simulink model "PCS_pu_DCDC"  (R2024a)
settings: Solver=FixedStepAuto  StartTime=0.0  StopTime=3  RelTol=1e-3
undefined symbols (not defined in the file or in its folder): DiscIntNeverNeededParam, initial
libraries: spsCurrentMeasurementLib x18, spsVoltageMeasurementLib x13, spsControlledVoltageSourceLib x9, spsSeriesRLCBranchLib x7, spsThreePhaseSeriesRLCBranchLib x5, slpidlib x4, spsGroundLib x2, spsControlledCurrentSourceLib x2, SimplusGT x2, spspowerguiLib x2
(part 2 of 2)

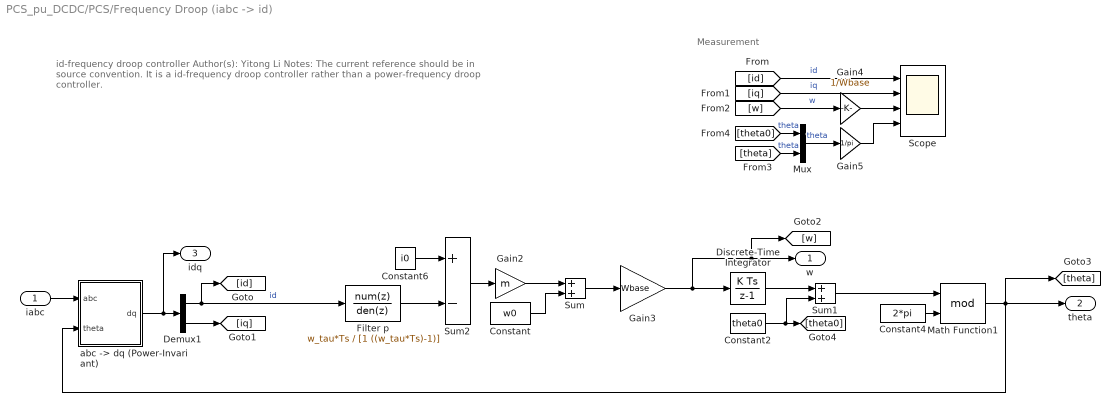
== system PCS_pu_DCDC/PCS/Frequency Droop (iabc -> id) ==
  note: Measurement
  note: id-frequency droop controller
      |
      | Author(s): Yitong Li
      |
      | Notes:
      |
      | The current reference should be in source convention.
      |
      | It is a id-frequency droop controller rather than a power-frequency droop controller.
  iabc : Inport
  Constant : Constant  Value=w0
  Constant2 : Constant  Value=theta0
  Constant4 : Constant  Value=2*pi
  Constant6 : Constant  Value=i0
  Demux1 : Demux  Outputs=2
  Discrete-Time Integrator : DiscreteIntegrator  SampleTime=Ts  ICPrevOutput=DiscIntNeverNeededParam  ICPrevScaledInput=DiscIntNeverNeededParam
  Filter p : DiscreteTransferFcn  Numerator=w_tau*Ts  Denominator=[1 ((w_tau*Ts)-1)]  SampleTime=Ts
  Gain2 : Gain  Gain=m
  Gain3 : Gain  Gain=Wbase
  Gain4 : Gain  Gain=1/Wbase
  Gain5 : Gain  Gain=1/pi
  Math Function1 : Math  Operator=mod  SignedPower=on
  Mux : Mux  Inputs=2
  Scope : Scope  NumInputPorts=4
  Sum : Sum
  Sum1 : Sum
  Sum2 : Sum  Inputs=+-
  "abc -> dq (Power-Invariant)" : Subsystem  AncestorBlock=|
      | SimplusGT/abc -> dq
      | (Power-Invariant)
  w : Outport
  theta : Outport  Port=2
  idq : Outport  Port=3
  wires:
  Sum1/1 -> Math Function1/1
  Constant2/1 -> Sum1/2, [theta0]
  Math Function1/1 -> "abc -> dq (Power-Invariant)"/2(theta), [theta], theta/1
  Gain2/1 -> Sum/1
  Discrete-Time Integrator/1 -> Sum1/1
  Filter p/1 -> Sum2/2
  Constant/1 -> Sum/2
  "abc -> dq (Power-Invariant)"/1(dq) -> idq/1, Demux1/1
  Constant4/1 -> Math Function1/2
  iabc/1 -> "abc -> dq (Power-Invariant)"/1(abc)
  Constant6/1 -> Sum2/1
  Sum2/1 -> Gain2/1
  Sum/1 -> Gain3/1
  Gain3/1 -> [w], w/1, Discrete-Time Integrator/1
  Demux1/1 -> [id], Filter p/1  "id"
  Gain5/1 -> Scope/4
  [iq] -> Scope/2  "iq"
  [theta0] -> Mux/1  "theta"
  [id] -> Scope/1  "id"
  Mux/1 -> Gain5/1  "theta"
  [theta] -> Mux/2  "theta"
  Demux1/2 -> [iq]
  [w] -> Gain4/1  "w"
  Gain4/1 -> Scope/3

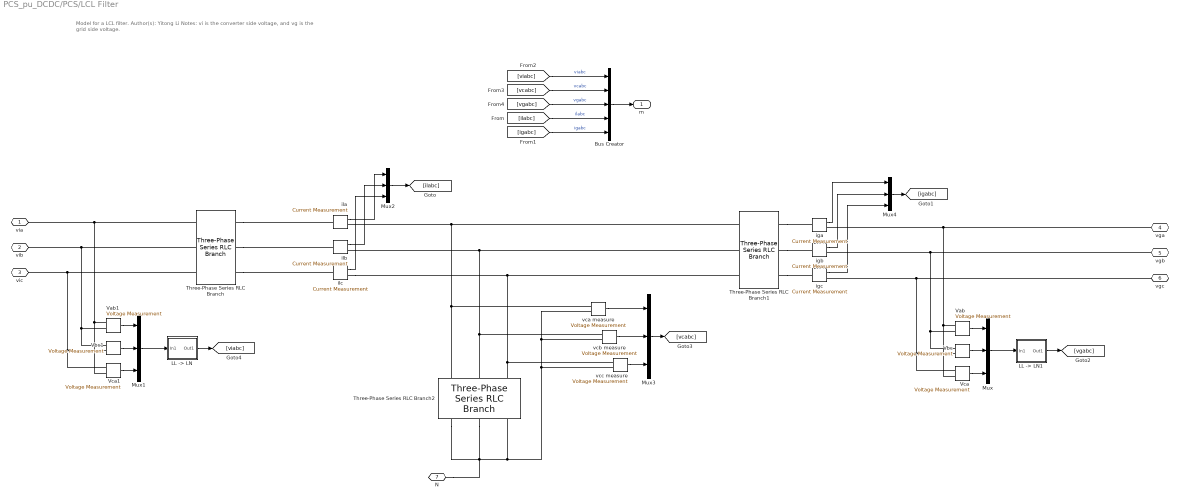
== system PCS_pu_DCDC/PCS/LCL Filter ==
  note: Model for a LCL filter.
      |
      | Author(s): Yitong Li
      |
      | Notes:
      |
      | vi is the converter side voltage, and vg is the grid side voltage.
  Bus Creator : BusCreator  Inputs=5
  "LL -> LN" : Subsystem  AncestorBlock=SimplusGT/LL -> LN
  "LL -> LN1" : Subsystem  AncestorBlock=|
      | SimplusGT/Grid-Forming Inverter
      | (Simulink Block)/LCL Filter/LL -> LN
  Mux{,1..4} (5 alike) : Mux  Inputs=3
  Three-Phase Series RLC Branch : spsThreePhaseSeriesRLCBranchLib/Three-Phase Series RLC Branch  LConnTagsString=A|B|C  RConnTagsString=A|B|C  BranchType=RL  Resistance=Rf  Inductance=Lf  Capacitance=1e-6  Measurements=None
  Three-Phase Series RLC Branch1 : spsThreePhaseSeriesRLCBranchLib/Three-Phase Series RLC Branch  LConnTagsString=A|B|C  RConnTagsString=A|B|C  BranchType=RL  Resistance=Rc  Inductance=Lc  Capacitance=1e-6  Measurements=None
  Three-Phase Series RLC Branch2 : spsThreePhaseSeriesRLCBranchLib/Three-Phase Series RLC Branch  LConnTagsString=A|B|C  RConnTagsString=A|B|C  BranchType=RC  Resistance=Rd  Inductance=Lc  Capacitance=Cf  Measurements=None
  Vab : spsVoltageMeasurementLib/Voltage Measurement  PhasorSimulation=off  OutputType=Complex  PSBequivalent=0
  Vab1 : spsVoltageMeasurementLib/Voltage Measurement  PhasorSimulation=off  OutputType=Complex  PSBequivalent=0
  Vbc : spsVoltageMeasurementLib/Voltage Measurement  PhasorSimulation=off  OutputType=Complex  PSBequivalent=0
  Vbc1 : spsVoltageMeasurementLib/Voltage Measurement  PhasorSimulation=off  OutputType=Complex  PSBequivalent=0
  Vca : spsVoltageMeasurementLib/Voltage Measurement  PhasorSimulation=off  OutputType=Complex  PSBequivalent=0
  Vca1 : spsVoltageMeasurementLib/Voltage Measurement  PhasorSimulation=off  OutputType=Complex  PSBequivalent=0
  iga : spsCurrentMeasurementLib/Current Measurement  PhasorSimulation=off  OutputType=Complex  PSBequivalent=0
  igb : spsCurrentMeasurementLib/Current Measurement  PhasorSimulation=off  OutputType=Complex  PSBequivalent=0
  igc : spsCurrentMeasurementLib/Current Measurement  PhasorSimulation=off  OutputType=Complex  PSBequivalent=0
  ila : spsCurrentMeasurementLib/Current Measurement  PhasorSimulation=off  OutputType=Complex  PSBequivalent=0
  ilb : spsCurrentMeasurementLib/Current Measurement  PhasorSimulation=off  OutputType=Complex  PSBequivalent=0
  ilc : spsCurrentMeasurementLib/Current Measurement  PhasorSimulation=off  OutputType=Complex  PSBequivalent=0
  vca measure : spsVoltageMeasurementLib/Voltage Measurement  PhasorSimulation=off  OutputType=Complex  PSBequivalent=0
  vcb measure : spsVoltageMeasurementLib/Voltage Measurement  PhasorSimulation=off  OutputType=Complex  PSBequivalent=0
  vcc measure : spsVoltageMeasurementLib/Voltage Measurement  PhasorSimulation=off  OutputType=Complex  PSBequivalent=0
  via : PMIOPort  Side=Left
  vib : PMIOPort  Port=2  Side=Left
  vic : PMIOPort  Port=3  Side=Left
  vga : PMIOPort  Port=4  Side=Right
  vgb : PMIOPort  Port=5  Side=Right
  vgc : PMIOPort  Port=6  Side=Right
  N : PMIOPort  Port=7  Side=Left
  m : Outport
  wires:
  Mux4/1 -> [igabc]
  ilb/1 -> Mux2/2
  ila/1 -> Mux2/1
  igc/1 -> Mux4/3
  vcc measure/1 -> Mux3/3
  Vab/1 -> Mux/1
  Mux/1 -> "LL -> LN1"/1(In1)
  vca measure/1 -> Mux3/1
  vcb measure/1 -> Mux3/2
  igb/1 -> Mux4/2
  iga/1 -> Mux4/1
  Vca/1 -> Mux/3
  ilc/1 -> Mux2/3
  Vbc/1 -> Mux/2
  Mux2/1 -> [ilabc]
  Bus Creator/1 -> m/1
  "LL -> LN1"/1(Out1) -> [vgabc]
  Mux3/1 -> [vcabc]
  Vbc1/1 -> Mux1/2
  Vca1/1 -> Mux1/3
  Mux1/1 -> "LL -> LN"/1(In1)
  Vab1/1 -> Mux1/1
  "LL -> LN"/1(Out1) -> [viabc]
  [viabc] -> Bus Creator/1  "viabc"
  [vcabc] -> Bus Creator/2  "vcabc"
  [vgabc] -> Bus Creator/3  "vgabc"
  [ilabc] -> Bus Creator/4  "ilabc"
  [igabc] -> Bus Creator/5  "igabc"
  connections:
  Three-Phase Series RLC Branch2/RConn1 -- Three-Phase Series RLC Branch2/RConn2 -- N/RConn1 -- Three-Phase Series RLC Branch2/RConn3 -- vcc measure/LConn2 -- vca measure/LConn2 -- vcb measure/LConn2
  Vca/LConn1 -- Vbc/LConn2 -- igc/RConn1 -- vgc/RConn1
  Vca1/LConn1 -- Vbc1/LConn2 -- vic/RConn1 -- Three-Phase Series RLC Branch/LConn3
  Three-Phase Series RLC Branch/LConn2 -- Vbc1/LConn1 -- Vab1/LConn2 -- vib/RConn1
  Vab1/LConn1 -- Vca1/LConn2 -- via/RConn1 -- Three-Phase Series RLC Branch/LConn1
  Three-Phase Series RLC Branch1/LConn3 -- ilc/RConn1 -- Three-Phase Series RLC Branch2/LConn3 -- vcc measure/LConn1
  Three-Phase Series RLC Branch1/RConn2 -- igb/LConn1
  Vbc/LConn1 -- Vab/LConn2 -- igb/RConn1 -- vgb/RConn1
  ilb/RConn1 -- Three-Phase Series RLC Branch1/LConn2 -- vcb measure/LConn1 -- Three-Phase Series RLC Branch2/LConn2
  ila/RConn1 -- Three-Phase Series RLC Branch1/LConn1 -- vca measure/LConn1 -- Three-Phase Series RLC Branch2/LConn1
  Vab/LConn1 -- Vca/LConn2 -- iga/RConn1 -- vga/RConn1
  Three-Phase Series RLC Branch1/RConn1 -- iga/LConn1
  Three-Phase Series RLC Branch1/RConn3 -- igc/LConn1
  Three-Phase Series RLC Branch/RConn1 -- ila/LConn1
  Three-Phase Series RLC Branch/RConn2 -- ilb/LConn1
  Three-Phase Series RLC Branch/RConn3 -- ilc/LConn1

== system PCS_pu_DCDC/PCS/PQ Calculation (dq-Frame) ==
  note: Power calculation.
      |
      | Author(s): Yitong Li
      |
      | Notes:
      |
      | The calculation is done in dq frame.
  vdq : Inport
  idq : Inport  Port=2
  Mux : Mux  Inputs=2
  Mux1 : Mux  Inputs=2
  P = vd*id+vq*iq : Fcn  Expr=u[1]*u[3]+u[2]*u[4]
  Q = -vd*iq+vq*id : Fcn  Expr=-u[1]*u[4]+u[2]*u[3]
  pq : Outport
  wires:
  Q = -vd*iq+vq*id/1 -> Mux/2
  Mux1/1 -> Q = -vd*iq+vq*id/1, P = vd*id+vq*iq/1
  idq/1 -> Mux1/2
  vdq/1 -> Mux1/1
  P = vd*id+vq*iq/1 -> Mux/1
  Mux/1 -> pq/1

== system PCS_pu_DCDC/PCS/SC_Voltage_controller ==
  vdc : Inport
  vdc_ref : Inport  Port=2
  Add : Sum  Inputs=+-
  Discrete PID Controller : slpidlib/PID Controller  Controller=PID  Form=Parallel  TimeDomain=Discrete-time  UseExternalTs=off  SampleTime=-1  IntegratorMethod=Forward Euler  FilterMethod=Forward Euler  ControllerParametersSource=internal  P=w_v*C  I=w_v*w_v*C/4  UseKiTs=off  D=0  UseExternalDerivativeSource=off  N=100  UseFilter=off  TunerSelectOption=Transfer Function Based (PID Tuner App)  InitialConditionSource=internal  InitialConditionForIntegrator=0  InitialConditionForFilter=0  DifferentiatorICPrevScaledInput=0  ExternalReset=none  TrackingMode=off  Kt=1  LimitOutput=off  SatLimitsSource=internal  UpperSaturationLimit=inf  LowerSaturationLimit=-inf  LinearizeAsGain=off  AntiWindupMode=none  Kb=1  LimitIntegrator=off  UpperIntegratorSaturationLimit=inf  LowerIntegratorSaturationLimit=-inf  POutMin=[]  POutMax=[]  IOutMin=[]  IOutMax=[]  DOutMin=[]  DOutMax=[]  NOutMin=[]  NOutMax=[]  SumOutMin=[]  SumOutMax=[]  SaturationOutMin=[]  SaturationOutMax=[]  PParamMin=[]  PParamMax=[]  IParamMin=[]  IParamMax=[]  DParamMin=[]  DParamMax=[]  NParamMin=[]  NParamMax=[]  KbParamMin=[]  KbParamMax=[]  KtParamMin=[]  KtParamMax=[]  KbOutMin=[]  KbOutMax=[]  KtOutMin=[]  KtOutMax=[]  IntegratorOutMin=[]  IntegratorOutMax=[]  FilterOutMin=[]  FilterOutMax=[]  SumI1OutMin=[]  SumI1OutMax=[]  SumI2OutMin=[]  SumI2OutMax=[]  SumI3OutMin=[]  SumI3OutMax=[]  SumI4OutMin=[]  SumI4OutMax=[]  SumDOutMin=[]  SumDOutMax=[]  DifferentiatorOutMin=[]  DifferentiatorOutMax=[]  FilterDiffOutCoefMin=[]  FilterDiffOutCoefMax=[]  ReciprocalOutMin=[]  ReciprocalOutMax=[]  SumDenOutMin=[]  SumDenOutMax=[]  SumNumOutMin=[]  SumNumOutMax=[]  DivideOutMin=[]  DivideOutMax=[]  UdiffTsProdOutMin=[]  UdiffTsProdOutMax=[]  NTsProdOutMin=[]  NTsProdOutMax=[]  UintegralTsProdOutMin=[]  UintegralTsProdOutMax=[]  UngainTsProdOutMin=[]  UngainTsProdOutMax=[]  ClampingZeroOutDataTypeStr=Inherit: Inherit via back propagation  ClampingZeroOutMin=[]  ClampingZeroOutMax=[]  FilterDenConstantOutDataTypeStr=Inherit: Inherit via back propagation  FilterDenConstantOutMin=[]  FilterDenConstantOutMax=[]  PCopyOutDataTypeStr=Inherit: Inherit via back propagation  PCopyOutMin=[]  PCopyOutMax=[]  NCopyOutDataTypeStr=Inherit: Inherit via back propagation  NCopyOutMin=[]  NCopyOutMax=[]  IntegratorContinuousStateAttributes=''  IntegratorStateMustResolveToSignalObject=off  IntegratorRTWStateStorageClass=Auto  FilterContinuousStateAttributes=''  FilterStateMustResolveToSignalObject=off  FilterRTWStateStorageClass=Auto  ParallelPVariant=InternalParameters  IdealPVariant=Disabled  IVariant=InternalParameters  DVariant=InternalParameters  IntegratorVariant=Discrete  SatVariant=Disabled  AWVariant=Passthrough  PCopyVariant=Disabled  TRVariant=Disabled  FdbkBlocksVariant=Forward  IdealPFdbkVariant=Disabled  SatFdbkVariant=Disabled  DerivativeFilterVariant=Differentiator  NVariant=Passthrough  NCopyVariant=Disabled_SignalSpec  FilterICVariant=InternalICsDifferentiator  IntegratorICVariant=InternalICs  ExternalResetVariant=Disabled  TRSumVariant=Passthrough  SumFdbkVariant=Disabled  SumVariant=Sum_PID  TsampFilterVariant=InternalTs  TsampNgainVariant=Passthrough  TsampIntegralVariant=Disabled_SignalSpec  ExternalSaturationOutDataTypeStr=Inherit: Same as second input  DerivativeSourceVariant=ErrorSignal
      settings: LibrarySourceBlock=simulink/Discrete/Discrete PID Controller
  Display : Display
  Display1 : Display
  i_ref : Outport
  wires:
  vdc_ref/1 -> Add/1
  vdc/1 -> Add/2
  Add/1 -> Display/1, Discrete PID Controller/1
  Discrete PID Controller/1 -> Display1/1, i_ref/1

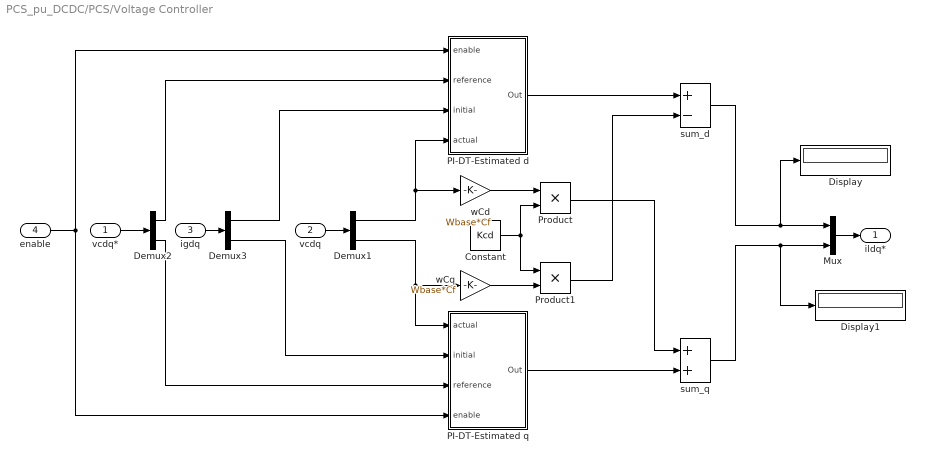
== system PCS_pu_DCDC/PCS/Voltage Controller ==
  vcdq* : Inport
  vcdq : Inport  Port=2
  igdq : Inport  Port=3
  enable : Inport  Port=4
  Constant : Constant  Value=Kcd
  Demux1 : Demux  Outputs=2
  Demux2 : Demux  Outputs=2
  Demux3 : Demux  Outputs=2
  Display : Display
  Display1 : Display
  Mux : Mux  Inputs=2
  PI-DT-Estimated d : Subsystem  mask{Kg=Kg, Kp=Kp, Ki=Ki, xmax=xdmax, xmin=-xdmax, Ts=Ts}
      mask prompts: Kg "Estimator Gain"; Kp "Proportional Gain"; Ki "Integral Gain"; xmax "Upper Limit"; xmin "Lower Limit"; Ts "Sampling Time"
  PI-DT-Estimated q : Subsystem  mask{Kg=Kg, Kp=Kp, Ki=Ki, xmax=xqmax, xmin=-xqmax, Ts=Ts}
      mask prompts: Kg "Estimator Gain"; Kp "Proportional Gain"; Ki "Integral Gain"; xmax "Upper Limit"; xmin "Lower Limit"; Ts "Sampling Time"
  Product : Product
  Product1 : Product
  sum_d : Sum  Inputs=+-
  sum_q : Sum
  wCd : Gain  Gain=Wbase*Cf
  wCq : Gain  Gain=Wbase*Cf
  ildq* : Outport
  wires:
  Constant/1 -> Product1/1, Product/2
  Product1/1 -> sum_d/2
  wCq/1 -> Product1/2
  Product/1 -> sum_q/1
  wCd/1 -> Product/1
  enable/1 -> PI-DT-Estimated d/1(enable), PI-DT-Estimated q/4(enable)
  Demux2/2 -> PI-DT-Estimated q/3(reference)
  Demux2/1 -> PI-DT-Estimated d/2(reference)
  vcdq*/1 -> Demux2/1
  Demux3/1 -> PI-DT-Estimated d/3(initial)
  Demux3/2 -> PI-DT-Estimated q/2(initial)
  PI-DT-Estimated q/1(Out) -> sum_q/2
  igdq/1 -> Demux3/1
  PI-DT-Estimated d/1(Out) -> sum_d/1
  Mux/1 -> ildq*/1
  Demux1/2 -> wCq/1, PI-DT-Estimated q/1(actual)
  Demux1/1 -> PI-DT-Estimated d/4(actual), wCd/1
  vcdq/1 -> Demux1/1
  sum_q/1 -> Display1/1, Mux/2
  sum_d/1 -> Display/1, Mux/1

== system PCS_pu_DCDC/PCS/abc -> dq (Power-Invariant) ==
  note: Frame transformation from abc to dq.
      |
      | Author(s): Yitong Li
      |
      | Notes:
      |
      | The transformation is power-invariant.
      |
      | theta is the angle that d axis leads a axis.
      |
      | q axis leads d axis by 90 degrees.
  abc : Inport
  theta : Inport  Port=2
  ->d : Fcn  Expr=cos(u(4))*u(1) + cos(u(4)-2/3*pi)*u(2) + cos(u(4)-4/3*pi)*u(3)
  ->q : Fcn  Expr=-sin(u(4))*u(1) - sin(u(4)-2/3*pi)*u(2) - sin(u(4)-4/3*pi)*u(3)
  Gain : Gain  Gain=sqrt(2/3)
  Mux5 : Mux  Inputs=2
  Mux6 : Mux  Inputs=2
  dq : Outport
  wires:
  Mux5/1 -> ->q/1, ->d/1
  Mux6/1 -> dq/1
  ->q/1 -> Mux6/2
  theta/1 -> Mux5/2
  Gain/1 -> Mux5/1
  ->d/1 -> Mux6/1
  abc/1 -> Gain/1

== system PCS_pu_DCDC/PCS/abc -> dq (Power-Invariant)1 ==
  note: Frame transformation from abc to dq.
      |
      | Author(s): Yitong Li
      |
      | Notes:
      |
      | The transformation is power-invariant.
      |
      | theta is the angle that d axis leads a axis.
      |
      | q axis leads d axis by 90 degrees.
  abc : Inport
  theta : Inport  Port=2
  ->d : Fcn  Expr=cos(u(4))*u(1) + cos(u(4)-2/3*pi)*u(2) + cos(u(4)-4/3*pi)*u(3)
  ->q : Fcn  Expr=-sin(u(4))*u(1) - sin(u(4)-2/3*pi)*u(2) - sin(u(4)-4/3*pi)*u(3)
  Gain : Gain  Gain=sqrt(2/3)
  Mux5 : Mux  Inputs=2
  Mux6 : Mux  Inputs=2
  dq : Outport
  wires:
  Mux5/1 -> ->q/1, ->d/1
  Mux6/1 -> dq/1
  ->q/1 -> Mux6/2
  theta/1 -> Mux5/2
  Gain/1 -> Mux5/1
  ->d/1 -> Mux6/1
  abc/1 -> Gain/1

== system PCS_pu_DCDC/PCS/abc -> dq (Power-Invariant)2 ==
  note: Frame transformation from abc to dq.
      |
      | Author(s): Yitong Li
      |
      | Notes:
      |
      | The transformation is power-invariant.
      |
      | theta is the angle that d axis leads a axis.
      |
      | q axis leads d axis by 90 degrees.
  abc : Inport
  theta : Inport  Port=2
  ->d : Fcn  Expr=cos(u(4))*u(1) + cos(u(4)-2/3*pi)*u(2) + cos(u(4)-4/3*pi)*u(3)
  ->q : Fcn  Expr=-sin(u(4))*u(1) - sin(u(4)-2/3*pi)*u(2) - sin(u(4)-4/3*pi)*u(3)
  Gain : Gain  Gain=sqrt(2/3)
  Mux5 : Mux  Inputs=2
  Mux6 : Mux  Inputs=2
  dq : Outport
  wires:
  Mux5/1 -> ->q/1, ->d/1
  Mux6/1 -> dq/1
  ->q/1 -> Mux6/2
  theta/1 -> Mux5/2
  Gain/1 -> Mux5/1
  ->d/1 -> Mux6/1
  abc/1 -> Gain/1

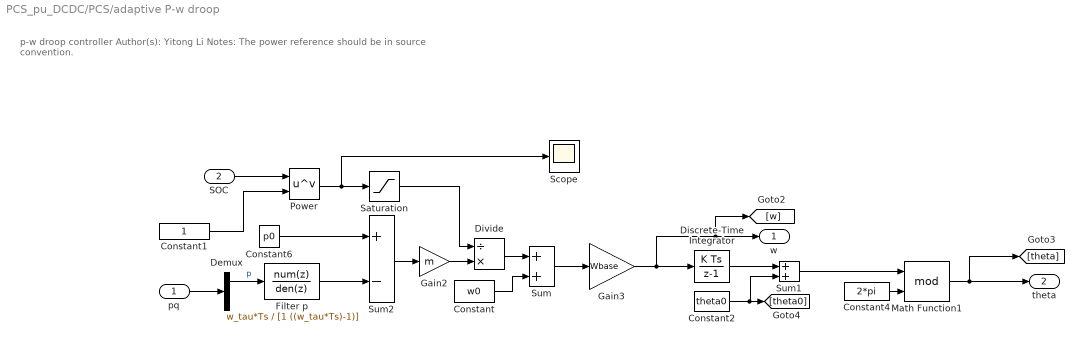
== system PCS_pu_DCDC/PCS/adaptive P-w droop ==
  note: p-w droop controller
      |
      | Author(s): Yitong Li
      |
      | Notes:
      |
      | The power reference should be in source convention.
  pq : Inport
  SOC : Inport  Port=2
  Constant : Constant  Value=w0
  Constant1 : Constant
  Constant2 : Constant  Value=theta0
  Constant4 : Constant  Value=2*pi
  Constant6 : Constant  Value=p0
  Demux : Demux  Outputs=2
  Discrete-Time Integrator : DiscreteIntegrator  SampleTime=Ts  ICPrevOutput=DiscIntNeverNeededParam  ICPrevScaledInput=DiscIntNeverNeededParam
  Divide : Product  Inputs=/*
  Filter p : DiscreteTransferFcn  Numerator=w_tau*Ts  Denominator=[1 ((w_tau*Ts)-1)]  SampleTime=Ts
  Gain2 : Gain  Gain=m
  Gain3 : Gain  Gain=Wbase
  Math Function1 : Math  Operator=mod  SignedPower=on
  Power : Math  Operator=pow
  Saturation : Saturate  UpperLimit=1  LowerLimit=0.1
  Scope : Scope
  Sum : Sum
  Sum1 : Sum
  Sum2 : Sum  Inputs=+-
  w : Outport
  theta : Outport  Port=2
  wires:
  Demux/1 -> Filter p/1  "p"
  Sum1/1 -> Math Function1/1
  Constant2/1 -> Sum1/2, [theta0]
  Math Function1/1 -> [theta], theta/1
  Discrete-Time Integrator/1 -> Sum1/1
  Filter p/1 -> Sum2/2
  Constant/1 -> Sum/2
  Constant4/1 -> Math Function1/2
  pq/1 -> Demux/1
  Constant6/1 -> Sum2/1
  Sum2/1 -> Gain2/1
  Sum/1 -> Gain3/1
  Gain3/1 -> [w], w/1, Discrete-Time Integrator/1
  Gain2/1 -> Divide/2
  Divide/1 -> Sum/1
  Saturation/1 -> Divide/1
  SOC/1 -> Power/1
  Power/1 -> Scope/1, Saturation/1
  Constant1/1 -> Power/2

== system PCS_pu_DCDC/PCS/dq -> abc (Power-Invariant) ==
  note: Frame transformation from dq to abc.
      |
      | Author(s): Yitong Li
      |
      | Notes:
      |
      | The transformation is power-invariant.
      |
      | theta is the angle that dq axis leads alpha/beta axis, specifically, d axis leads alpha axis.
  dq : Inport
  theta : Inport  Port=2
  ->a : Fcn  Expr=cos(u(3))*u(1) - sin(u(3))*u(2)
  ->b : Fcn  Expr=cos(u(3)-2/3*pi)*u(1) - sin(u(3)-2/3*pi)*u(2)
  ->c : Fcn  Expr=cos(u(3)-4/3*pi)*u(1) - sin(u(3)-4/3*pi)*u(2)
  Gain : Gain  Gain=sqrt(2/3)
  Mux5 : Mux  Inputs=2
  Mux6 : Mux  Inputs=3
  abc : Outport
  wires:
  theta/1 -> Mux5/2
  Mux5/1 -> ->c/1, ->a/1, ->b/1
  Mux6/1 -> abc/1
  ->c/1 -> Mux6/3
  dq/1 -> Gain/1
  Gain/1 -> Mux5/1
  ->a/1 -> Mux6/1
  ->b/1 -> Mux6/2

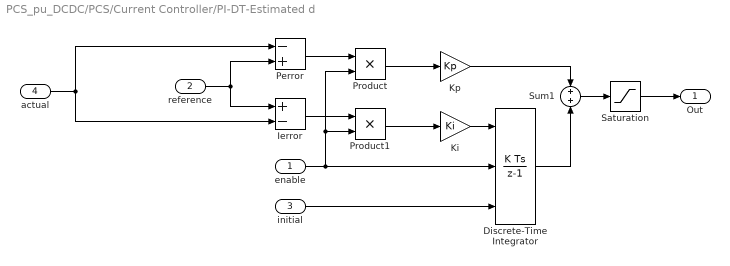
== system PCS_pu_DCDC/PCS/Current Controller/PI-DT-Estimated d ==
  enable : Inport
  reference : Inport  Port=2
  initial : Inport  Port=3
  actual : Inport  Port=4
  Discrete-Time Integrator : DiscreteIntegrator  gainval=1  ExternalReset=rising  InitialConditionSource=external  InitialCondition=initial  SampleTime=Ts  LimitOutput=on  UpperSaturationLimit=xmax  LowerSaturationLimit=xmin  ICPrevOutput=DiscIntNeverNeededParam  ICPrevScaledInput=DiscIntNeverNeededParam
  Ierror : Sum  Inputs=+-
  Ki : Gain  Gain=Ki  SaturateOnIntegerOverflow=on  OutDataTypeStr=Inherit: Same as input  ParamDataTypeStr=Inherit: Same as input
  Kp : Gain  Gain=Kp  SaturateOnIntegerOverflow=on  OutDataTypeStr=Inherit: Same as input  ParamDataTypeStr=Inherit: Same as input
  Perror : Sum  Inputs=-+
  Product : Product  RndMeth=Zero
  Product1 : Product  RndMeth=Zero
  Saturation : Saturate  UpperLimit=xmax  LowerLimit=xmin
  Sum1 : Sum  SaturateOnIntegerOverflow=on
  Out : Outport
  wires:
  Product1/1 -> Ki/1
  Ierror/1 -> Product1/1
  Product/1 -> Kp/1
  Perror/1 -> Product/1
  reference/1 -> Ierror/1, Perror/2
  actual/1 -> Ierror/2, Perror/1
  initial/1 -> Discrete-Time Integrator/3
  enable/1 -> Product1/2, Product/2, Discrete-Time Integrator/2
  Discrete-Time Integrator/1 -> Sum1/2
  Kp/1 -> Sum1/1
  Ki/1 -> Discrete-Time Integrator/1
  Sum1/1 -> Saturation/1
  Saturation/1 -> Out/1

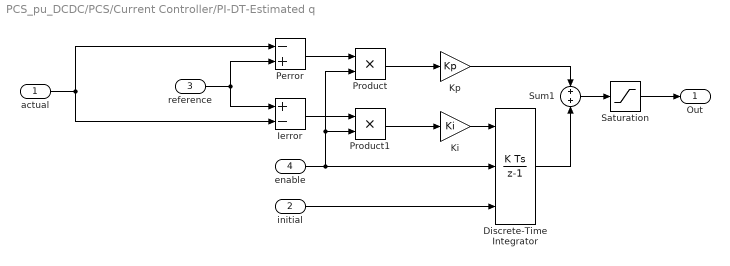
== system PCS_pu_DCDC/PCS/Current Controller/PI-DT-Estimated q ==
  actual : Inport
  initial : Inport  Port=2
  reference : Inport  Port=3
  enable : Inport  Port=4
  Discrete-Time Integrator : DiscreteIntegrator  gainval=1  ExternalReset=rising  InitialConditionSource=external  InitialCondition=initial  SampleTime=Ts  LimitOutput=on  UpperSaturationLimit=xmax  LowerSaturationLimit=xmin  ICPrevOutput=DiscIntNeverNeededParam  ICPrevScaledInput=DiscIntNeverNeededParam
  Ierror : Sum  Inputs=+-
  Ki : Gain  Gain=Ki  SaturateOnIntegerOverflow=on  OutDataTypeStr=Inherit: Same as input  ParamDataTypeStr=Inherit: Same as input
  Kp : Gain  Gain=Kp  SaturateOnIntegerOverflow=on  OutDataTypeStr=Inherit: Same as input  ParamDataTypeStr=Inherit: Same as input
  Perror : Sum  Inputs=-+
  Product : Product  RndMeth=Zero
  Product1 : Product  RndMeth=Zero
  Saturation : Saturate  UpperLimit=xmax  LowerLimit=xmin
  Sum1 : Sum  SaturateOnIntegerOverflow=on
  Out : Outport
  wires:
  Product1/1 -> Ki/1
  Ierror/1 -> Product1/1
  Product/1 -> Kp/1
  Perror/1 -> Product/1
  reference/1 -> Ierror/1, Perror/2
  actual/1 -> Perror/1, Ierror/2
  initial/1 -> Discrete-Time Integrator/3
  enable/1 -> Product1/2, Product/2, Discrete-Time Integrator/2
  Discrete-Time Integrator/1 -> Sum1/2
  Kp/1 -> Sum1/1
  Ki/1 -> Discrete-Time Integrator/1
  Sum1/1 -> Saturation/1
  Saturation/1 -> Out/1

== system PCS_pu_DCDC/PCS/Frequency Droop (iabc -> id)/abc -> dq (Power-Invariant) ==
  note: Frame transformation from abc to dq.
      |
      | Author(s): Yitong Li
      |
      | Notes:
      |
      | The transformation is power-invariant.
      |
      | theta is the angle that d axis leads a axis.
      |
      | q axis leads d axis by 90 degrees.
  abc : Inport
  theta : Inport  Port=2
  ->d : Fcn  Expr=cos(u(4))*u(1) + cos(u(4)-2/3*pi)*u(2) + cos(u(4)-4/3*pi)*u(3)
  ->q : Fcn  Expr=-sin(u(4))*u(1) - sin(u(4)-2/3*pi)*u(2) - sin(u(4)-4/3*pi)*u(3)
  Gain : Gain  Gain=sqrt(2/3)
  Mux5 : Mux  Inputs=2
  Mux6 : Mux  Inputs=2
  dq : Outport
  wires:
  abc/1 -> Gain/1
  ->d/1 -> Mux6/1
  Gain/1 -> Mux5/1
  theta/1 -> Mux5/2
  ->q/1 -> Mux6/2
  Mux6/1 -> dq/1
  Mux5/1 -> ->d/1, ->q/1

== system PCS_pu_DCDC/PCS/LCL Filter/LL -> LN ==
  note: Transformation from line-to-line voltage to line-to-neutral voltage.
      |
      | Author(s): Yitong Li
  In1 : Inport
  Fcn : Fcn  Expr=u[1]-u[3]
  Fcn1 : Fcn  Expr=u[2]-u[1]
  Fcn2 : Fcn  Expr=u[3]-u[2]
  Gain : Gain  Gain=1/3
  Mux9 : Mux  Inputs=3
  Out1 : Outport
  wires:
  In1/1 -> Gain/1
  Gain/1 -> Fcn/1, Fcn1/1, Fcn2/1
  Mux9/1 -> Out1/1
  Fcn2/1 -> Mux9/3
  Fcn1/1 -> Mux9/2
  Fcn/1 -> Mux9/1

== system PCS_pu_DCDC/PCS/LCL Filter/LL -> LN1 ==
  note: Transformation from line-to-line voltage to line-to-neutral voltage.
      |
      | Author(s): Yitong Li
  In1 : Inport
  Fcn : Fcn  Expr=u[1]-u[3]
  Fcn1 : Fcn  Expr=u[2]-u[1]
  Fcn2 : Fcn  Expr=u[3]-u[2]
  Gain : Gain  Gain=1/3
  Mux9 : Mux  Inputs=3
  Out1 : Outport
  wires:
  In1/1 -> Gain/1
  Gain/1 -> Fcn/1, Fcn1/1, Fcn2/1
  Mux9/1 -> Out1/1
  Fcn2/1 -> Mux9/3
  Fcn1/1 -> Mux9/2
  Fcn/1 -> Mux9/1

== system PCS_pu_DCDC/PCS/Voltage Controller/PI-DT-Estimated d ==
  enable : Inport
  reference : Inport  Port=2
  initial : Inport  Port=3
  actual : Inport  Port=4
  Discrete-Time Integrator : DiscreteIntegrator  gainval=1  ExternalReset=rising  InitialConditionSource=external  InitialCondition=initial  SampleTime=Ts  LimitOutput=on  UpperSaturationLimit=xmax  LowerSaturationLimit=xmin  ICPrevOutput=DiscIntNeverNeededParam  ICPrevScaledInput=DiscIntNeverNeededParam
  Ierror : Sum  Inputs=+-
  Ki : Gain  Gain=Ki  SaturateOnIntegerOverflow=on  OutDataTypeStr=Inherit: Same as input  ParamDataTypeStr=Inherit: Same as input
  Kp : Gain  Gain=Kp  SaturateOnIntegerOverflow=on  OutDataTypeStr=Inherit: Same as input  ParamDataTypeStr=Inherit: Same as input
  Perror : Sum  Inputs=-+
  Product : Product  RndMeth=Zero
  Product1 : Product  RndMeth=Zero
  Saturation : Saturate  UpperLimit=xmax  LowerLimit=xmin
  Sum1 : Sum  SaturateOnIntegerOverflow=on
  Out : Outport
  wires:
  Product1/1 -> Ki/1
  Ierror/1 -> Product1/1
  Product/1 -> Kp/1
  Perror/1 -> Product/1
  reference/1 -> Ierror/1, Perror/2
  actual/1 -> Ierror/2, Perror/1
  initial/1 -> Discrete-Time Integrator/3
  enable/1 -> Product1/2, Product/2, Discrete-Time Integrator/2
  Discrete-Time Integrator/1 -> Sum1/2
  Kp/1 -> Sum1/1
  Ki/1 -> Discrete-Time Integrator/1
  Sum1/1 -> Saturation/1
  Saturation/1 -> Out/1

== system PCS_pu_DCDC/PCS/Voltage Controller/PI-DT-Estimated q ==
  actual : Inport
  initial : Inport  Port=2
  reference : Inport  Port=3
  enable : Inport  Port=4
  Discrete-Time Integrator : DiscreteIntegrator  gainval=1  ExternalReset=rising  InitialConditionSource=external  InitialCondition=initial  SampleTime=Ts  LimitOutput=on  UpperSaturationLimit=xmax  LowerSaturationLimit=xmin  ICPrevOutput=DiscIntNeverNeededParam  ICPrevScaledInput=DiscIntNeverNeededParam
  Ierror : Sum  Inputs=+-
  Ki : Gain  Gain=Ki  SaturateOnIntegerOverflow=on  OutDataTypeStr=Inherit: Same as input  ParamDataTypeStr=Inherit: Same as input
  Kp : Gain  Gain=Kp  SaturateOnIntegerOverflow=on  OutDataTypeStr=Inherit: Same as input  ParamDataTypeStr=Inherit: Same as input
  Perror : Sum  Inputs=-+
  Product : Product  RndMeth=Zero
  Product1 : Product  RndMeth=Zero
  Saturation : Saturate  UpperLimit=xmax  LowerLimit=xmin
  Sum1 : Sum  SaturateOnIntegerOverflow=on
  Out : Outport
  wires:
  Product1/1 -> Ki/1
  Ierror/1 -> Product1/1
  Product/1 -> Kp/1
  Perror/1 -> Product/1
  reference/1 -> Ierror/1, Perror/2
  actual/1 -> Perror/1, Ierror/2
  initial/1 -> Discrete-Time Integrator/3
  enable/1 -> Product1/2, Product/2, Discrete-Time Integrator/2
  Discrete-Time Integrator/1 -> Sum1/2
  Kp/1 -> Sum1/1
  Ki/1 -> Discrete-Time Integrator/1
  Sum1/1 -> Saturation/1
  Saturation/1 -> Out/1
